simulink model "ADRC1_PK_2RD"  (Simulink 7.6)
settings: Solver=ode45  StartTime=0.0  StopTime=1000  RelTol=1e-3
libraries: opclib x3, ADRC x1
settings Model: Creator=Administrator  LastModifiedBy=Administrator
settings DebuggingCC: SolverPrmCheckMsg=none

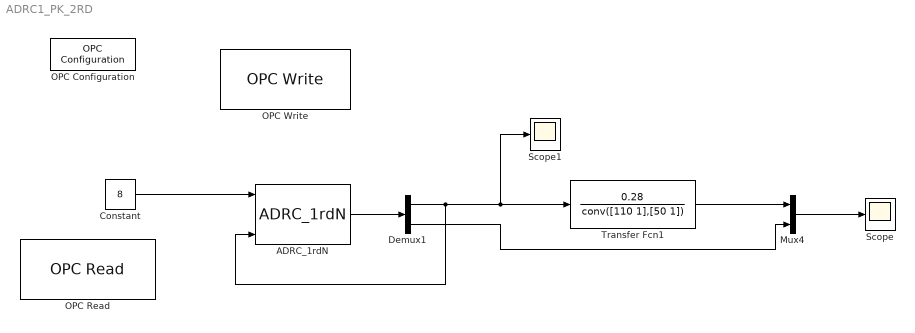
== system ADRC1_PK_2RD ==
  ADRC_1rdN : ADRC/ADRC/ADRC_1rd/ADRC_1rdN  SystemSampleTime=-1  RT=300  h=0.05  B01=30  B02=3000  r=0.01
  Constant : Constant  Value=8
  Demux1 : Demux  Outputs=2
  Mux4 : Mux  Inputs=2
  OPC Configuration : opclib/OPC Configuration  errMissingItems=Error  errReadWrite=Warn  errShutdown=Error  errRTViolation=Warn  rtEnable=on  speedup=1  showLatency=off  beingUsed=on
  OPC Read : opclib/OPC Read  readMode=Synchronous (cache)  dataType=double  updateRate=0.5  showQual=on  showTS=on  tsMode=Seconds since start
  OPC Write : opclib/OPC Write  writeMode=Synchronous  updateRate=0
  Scope : Scope
      settings: TimeRange=1000  YMin=0  YMax=12  DataFormat=Array
  Scope1 : Scope
      settings: TimeRange=1000  YMin=-2e+235  YMax=1.4e+236  DataFormat=Array
  Transfer Fcn1 : TransferFcn  Numerator=0.28  Denominator=conv([110 1],[50 1])
  wires:
  Constant/1 -> ADRC_1rdN/1
  ADRC_1rdN/1 -> Demux1/1
  Demux1/1 -> ADRC_1rdN/3, Transfer Fcn1/1, Scope1/1
  ? -> ?
  Transfer Fcn1/1 -> Mux4/1
  Demux1/2 -> Mux4/2
  Mux4/1 -> Scope/1
